simulink subsystem "Inverso"  (R2023b)
settings: Solver=VariableStepAuto  StartTime=0.0  StopTime=10.0  RelTol=1e-3
undefined symbols (not defined in the file): d
settings Model: Creator=Usuario  LastModifiedBy=Usuario_UMA

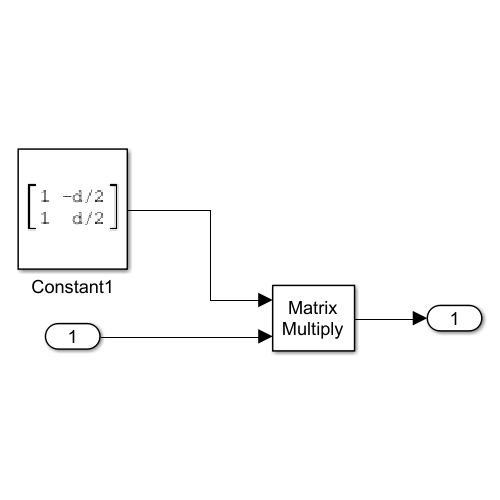
[thumbnail: Simulink's stored preview of the top-level diagram]
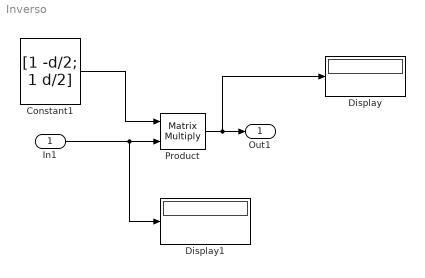
== system Inverso ==
  In1 : Inport
  Constant1 : Constant  Value=[1 -d/2; 1 d/2]  VectorParams1D=off  SampleTime=-1
  Display : Display
  Display1 : Display
  Product : Product  Multiplication=Matrix(*)
  Out1 : Outport
  wires:
  Constant1/1 -> Product/1
  Product/1 -> Out1/1, Display/1
  In1/1 -> Product/2, Display1/1
